simulink model "proyecto_4"  (R2021b)
settings: Solver=FixedStepDiscrete  StartTime=0.0  StopTime=Tsim  FixedStep=Tint  MaxStep=1e-6  RelTol=1e-6
InitFcn:
  | run init_fcn.m;
values from neighbouring files (symbols this model uses):
  C_init_v = 317    [init_fcn.m]
  C_load = 5e-2    (= 0.05)    [init_fcn.m]
  C_V = c_v * ro_air * volume_room    (= 220.63309632)    [init_fcn.m]
  Irr = 1000    [init_fcn.m]
  K_cond = Window_area * k_glass / esp    (= 158.4)    [init_fcn.m]
  L_s = 5e-3    (= 0.005)    [init_fcn.m]
  R_cuarto = 100    [init_fcn.m]
  shift = (180/3)/360 * Ts    (= 8.33333333333e-05)    [init_fcn.m]
  ss2 = c2d(ss2c, T_pred, 'tustin')    [init_fcn.m]
  T_ext = 15    [init_fcn.m]
  T_pred = Ts    (= 0.0005)    [init_fcn.m]
  Tint = 5e-5    (= 5e-05)    [init_fcn.m]
  Ts = 0.0005    [init_fcn.m]
  V_H4 = 300    [init_fcn.m]
  V_source = 230 * sqrt(2)    [init_fcn.m]
undefined symbols (not defined in the file or in its folder): DiscIntNeverNeededParam, F, K, Kobs, M, N, N2, Q, T_Enable, Temp_ref, Tsim, U0, X0
libraries: spsIGBTDiodeLib x17, spsVoltageMeasurementLib x11, simulink x8, spsCurrentMeasurementLib x8, slpidlib x6, spsSeriesRLCBranchLib x5, spsParallelRLCBranchLib x4, spsPVArrayLib x3, spsACVoltageSourceLib x1, spsDiodeLib x1, spspowerguiLib x1
(part 2 of 2)

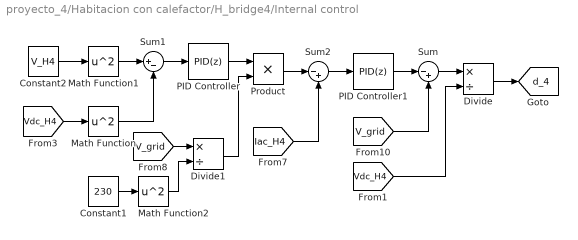
== system proyecto_4/Habitacion con calefactor/H_bridge4/Internal control ==
  Constant1 : Constant  Value=230
  Constant2 : Constant  Value=V_H4
  Divide : Product  Inputs=*/
  Divide1 : Product  Inputs=*/
  Math Function : Math  Operator=square  SaturateOnIntegerOverflow=on
  Math Function1 : Math  Operator=square  SaturateOnIntegerOverflow=on
  Math Function2 : Math  Operator=square  SaturateOnIntegerOverflow=on
  PID Controller : slpidlib/PID Controller  Controller=PID  Form=Parallel  TimeDomain=Discrete-time  UseExternalTs=off  SampleTime=Ts  IntegratorMethod=Forward Euler  FilterMethod=Forward Euler  ControllerParametersSource=internal  P=2  I=10  D=0  UseFilter=on  N=100  TunerSelectOption=Transfer Function Based (PID Tuner App)  InitialConditionSource=internal  InitialConditionForIntegrator=0  InitialConditionForFilter=0  DifferentiatorICPrevScaledInput=0  ExternalReset=none  TrackingMode=off  Kt=1  LimitOutput=off  SatLimitsSource=internal  UpperSaturationLimit=inf  LowerSaturationLimit=-inf  LinearizeAsGain=on  AntiWindupMode=none  Kb=1  POutMin=[]  POutMax=[]  IOutMin=[]  IOutMax=[]  DOutMin=[]  DOutMax=[]  NOutMin=[]  NOutMax=[]  SumOutMin=[]  SumOutMax=[]  SaturationOutMin=[]  SaturationOutMax=[]  PParamMin=[]  PParamMax=[]  IParamMin=[]  IParamMax=[]  DParamMin=[]  DParamMax=[]  NParamMin=[]  NParamMax=[]  KbParamMin=[]  KbParamMax=[]  KtParamMin=[]  KtParamMax=[]  KbOutMin=[]  KbOutMax=[]  KtOutMin=[]  KtOutMax=[]  IntegratorOutMin=[]  IntegratorOutMax=[]  FilterOutMin=[]  FilterOutMax=[]  SumI1OutMin=[]  SumI1OutMax=[]  SumI2OutMin=[]  SumI2OutMax=[]  SumI3OutMin=[]  SumI3OutMax=[]  SumI4OutMin=[]  SumI4OutMax=[]  SumDOutMin=[]  SumDOutMax=[]  DifferentiatorOutMin=[]  DifferentiatorOutMax=[]  FilterDiffOutCoefMin=[]  FilterDiffOutCoefMax=[]  ReciprocalOutMin=[]  ReciprocalOutMax=[]  SumDenOutMin=[]  SumDenOutMax=[]  SumNumOutMin=[]  SumNumOutMax=[]  DivideOutMin=[]  DivideOutMax=[]  UdiffTsProdOutMin=[]  UdiffTsProdOutMax=[]  NTsProdOutMin=[]  NTsProdOutMax=[]  UintegralTsProdOutMin=[]  UintegralTsProdOutMax=[]  UngainTsProdOutMin=[]  UngainTsProdOutMax=[]  IntegratorContinuousStateAttributes=''  IntegratorStateMustResolveToSignalObject=off  IntegratorRTWStateStorageClass=Auto  FilterContinuousStateAttributes=''  FilterStateMustResolveToSignalObject=off  FilterRTWStateStorageClass=Auto  ParallelPVariant=InternalParameters  IdealPVariant=Disabled  IVariant=InternalParameters  DVariant=InternalParameters  IntegratorVariant=Discrete  SatVariant=Disabled  AWVariant=Passthrough  PCopyVariant=Disabled  TRVariant=Disabled  FdbkBlocksVariant=Forward  IdealPFdbkVariant=Disabled  SatFdbkVariant=Disabled  DerivativeFilterVariant=ForwardEulerFilter  NVariant=InternalParameters  NCopyVariant=Disabled  FilterICVariant=InternalICsFilter  IntegratorICVariant=InternalICs  ExternalResetVariant=Disabled  TRSumVariant=Passthrough  SumFdbkVariant=Disabled  SumVariant=Sum_PID  TsampFilterVariant=InternalTs  TsampNgainVariant=Passthrough  TsampIntegralVariant=Passthrough  ExternalSaturationOutDataTypeStr=Inherit: Same as second input
  PID Controller1 : slpidlib/PID Controller  Controller=PID  Form=Parallel  TimeDomain=Discrete-time  UseExternalTs=off  SampleTime=Ts  IntegratorMethod=Forward Euler  FilterMethod=Forward Euler  ControllerParametersSource=internal  P=5  I=10  D=0  UseFilter=on  N=100  TunerSelectOption=Transfer Function Based (PID Tuner App)  InitialConditionSource=internal  InitialConditionForIntegrator=0  InitialConditionForFilter=0  DifferentiatorICPrevScaledInput=0  ExternalReset=none  TrackingMode=off  Kt=1  LimitOutput=off  SatLimitsSource=internal  UpperSaturationLimit=inf  LowerSaturationLimit=-inf  LinearizeAsGain=on  AntiWindupMode=none  Kb=1  POutMin=[]  POutMax=[]  IOutMin=[]  IOutMax=[]  DOutMin=[]  DOutMax=[]  NOutMin=[]  NOutMax=[]  SumOutMin=[]  SumOutMax=[]  SaturationOutMin=[]  SaturationOutMax=[]  PParamMin=[]  PParamMax=[]  IParamMin=[]  IParamMax=[]  DParamMin=[]  DParamMax=[]  NParamMin=[]  NParamMax=[]  KbParamMin=[]  KbParamMax=[]  KtParamMin=[]  KtParamMax=[]  KbOutMin=[]  KbOutMax=[]  KtOutMin=[]  KtOutMax=[]  IntegratorOutMin=[]  IntegratorOutMax=[]  FilterOutMin=[]  FilterOutMax=[]  SumI1OutMin=[]  SumI1OutMax=[]  SumI2OutMin=[]  SumI2OutMax=[]  SumI3OutMin=[]  SumI3OutMax=[]  SumI4OutMin=[]  SumI4OutMax=[]  SumDOutMin=[]  SumDOutMax=[]  DifferentiatorOutMin=[]  DifferentiatorOutMax=[]  FilterDiffOutCoefMin=[]  FilterDiffOutCoefMax=[]  ReciprocalOutMin=[]  ReciprocalOutMax=[]  SumDenOutMin=[]  SumDenOutMax=[]  SumNumOutMin=[]  SumNumOutMax=[]  DivideOutMin=[]  DivideOutMax=[]  UdiffTsProdOutMin=[]  UdiffTsProdOutMax=[]  NTsProdOutMin=[]  NTsProdOutMax=[]  UintegralTsProdOutMin=[]  UintegralTsProdOutMax=[]  UngainTsProdOutMin=[]  UngainTsProdOutMax=[]  IntegratorContinuousStateAttributes=''  IntegratorStateMustResolveToSignalObject=off  IntegratorRTWStateStorageClass=Auto  FilterContinuousStateAttributes=''  FilterStateMustResolveToSignalObject=off  FilterRTWStateStorageClass=Auto  ParallelPVariant=InternalParameters  IdealPVariant=Disabled  IVariant=InternalParameters  DVariant=InternalParameters  IntegratorVariant=Discrete  SatVariant=Disabled  AWVariant=Passthrough  PCopyVariant=Disabled  TRVariant=Disabled  FdbkBlocksVariant=Forward  IdealPFdbkVariant=Disabled  SatFdbkVariant=Disabled  DerivativeFilterVariant=ForwardEulerFilter  NVariant=InternalParameters  NCopyVariant=Disabled  FilterICVariant=InternalICsFilter  IntegratorICVariant=InternalICs  ExternalResetVariant=Disabled  TRSumVariant=Passthrough  SumFdbkVariant=Disabled  SumVariant=Sum_PID  TsampFilterVariant=InternalTs  TsampNgainVariant=Passthrough  TsampIntegralVariant=Passthrough  ExternalSaturationOutDataTypeStr=Inherit: Same as second input
  Product : Product
  Sum : Sum  Inputs=|-+
  Sum1 : Sum  Inputs=|+-
  Sum2 : Sum  Inputs=|-+
  tag scope: d_4=global
  wires:
  Divide/1 -> [d_4]
  Math Function1/1 -> Sum1/1
  [Iac_H4] -> Sum2/2
  Sum1/1 -> PID Controller/1
  Math Function/1 -> Sum1/2
  PID Controller1/1 -> Sum/1
  [Vdc_H4] -> Math Function/1
  PID Controller/1 -> Product/1
  Divide1/1 -> Product/2
  [V_grid] -> Sum/2
  Sum2/1 -> PID Controller1/1
  Sum/1 -> Divide/1
  [Vdc_H4] -> Divide/2
  Constant1/1 -> Math Function2/1
  [V_grid] -> Divide1/1
  Math Function2/1 -> Divide1/2
  Product/1 -> Sum2/1
  Constant2/1 -> Math Function1/1

== system proyecto_4/Habitacion con calefactor/H_bridge4/Measurements ==
  Current Measurement : spsCurrentMeasurementLib/Current Measurement  PhasorSimulation=off  OutputType=Complex  PSBequivalent=0
  V : spsVoltageMeasurementLib/Voltage Measurement  PhasorSimulation=off  OutputType=Complex  PSBequivalent=0
  in + : PMIOPort  Side=Left
  - : PMIOPort  Port=2  Side=Left
  out + : PMIOPort  Port=3  Side=Right
  -- : PMIOPort  Port=4  Side=Right
  tag scope: Iac_H4=global, Vac_H4=global
  wires:
  V/1 -> [Vac_H4]
  Current Measurement/1 -> [Iac_H4]
  connections:
  V/LConn2 -- --/RConn1 -- -/RConn1
  V/LConn1 -- Current Measurement/RConn1 -- out +/RConn1
  Current Measurement/LConn1 -- in +/RConn1

== system proyecto_4/Habitacion con calefactor/H_bridge4/Measurements1 ==
  Current Measurement : spsCurrentMeasurementLib/Current Measurement  PhasorSimulation=off  OutputType=Complex  PSBequivalent=0
  V : spsVoltageMeasurementLib/Voltage Measurement  PhasorSimulation=off  OutputType=Complex  PSBequivalent=0
  i + : PMIOPort  Side=Left
  i - : PMIOPort  Port=2  Side=Left
  o + : PMIOPort  Port=3  Side=Right
  o- : PMIOPort  Port=4  Side=Right
  tag scope: Idc_H4=global, Vdc_H4=global
  wires:
  V/1 -> [Vdc_H4]
  Current Measurement/1 -> [Idc_H4]
  connections:
  o-/RConn1 -- i -/RConn1 -- V/LConn2
  V/LConn1 -- o +/RConn1 -- Current Measurement/LConn1
  Current Measurement/RConn1 -- i +/RConn1

== system proyecto_4/H_bridge1/H_basic/Modulator2/Restriccion ==
  In1 : Inport
  In2 : Inport  Port=2
  Logical Operator1 : Logic  Operator=NOT  AllPortsSameDT=off  OutDataTypeStr=boolean
  Logical Operator2 : Logic  Operator=NOT  AllPortsSameDT=off  OutDataTypeStr=boolean
  Out1 : Outport
  Out2 : Outport  Port=2
  Out3 : Outport  Port=3
  Out4 : Outport  Port=4
  wires:
  In1/1 -> Out1/1, Logical Operator1/1
  In2/1 -> Out3/1, Logical Operator2/1
  Logical Operator2/1 -> Out4/1
  Logical Operator1/1 -> Out2/1

== system proyecto_4/H_bridge1/H_basic/Modulator2/Unipolar ==
  Duty : Inport
  Triag : Inport  Port=2
  Gain : Gain  Gain=-1
  Relational Operator : RelationalOperator  OutDataTypeStr=boolean  RndMeth=Simplest
  Relational Operator1 : RelationalOperator  OutDataTypeStr=boolean  RndMeth=Simplest
  Out1 : Outport
  Out2 : Outport  Port=2
  wires:
  Relational Operator/1 -> Out1/1
  Triag/1 -> Relational Operator/2, Gain/1
  Duty/1 -> Relational Operator1/2, Relational Operator/1
  Relational Operator1/1 -> Out2/1
  Gain/1 -> Relational Operator1/1

== system proyecto_4/H_bridge2/H_basic/Modulator2/Restriccion ==
  In1 : Inport
  In2 : Inport  Port=2
  Logical Operator1 : Logic  Operator=NOT  AllPortsSameDT=off  OutDataTypeStr=boolean
  Logical Operator2 : Logic  Operator=NOT  AllPortsSameDT=off  OutDataTypeStr=boolean
  Out1 : Outport
  Out2 : Outport  Port=2
  Out3 : Outport  Port=3
  Out4 : Outport  Port=4
  wires:
  In1/1 -> Out1/1, Logical Operator1/1
  In2/1 -> Out3/1, Logical Operator2/1
  Logical Operator2/1 -> Out4/1
  Logical Operator1/1 -> Out2/1

== system proyecto_4/H_bridge2/H_basic/Modulator2/Unipolar ==
  Duty : Inport
  Triag : Inport  Port=2
  Gain : Gain  Gain=-1
  Relational Operator : RelationalOperator  OutDataTypeStr=boolean  RndMeth=Simplest
  Relational Operator1 : RelationalOperator  OutDataTypeStr=boolean  RndMeth=Simplest
  Out1 : Outport
  Out2 : Outport  Port=2
  wires:
  Relational Operator/1 -> Out1/1
  Triag/1 -> Relational Operator/2, Gain/1
  Duty/1 -> Relational Operator1/2, Relational Operator/1
  Relational Operator1/1 -> Out2/1
  Gain/1 -> Relational Operator1/1

== system proyecto_4/H_bridge3/H_basic/Modulator2/Restriccion ==
  In1 : Inport
  In2 : Inport  Port=2
  Logical Operator1 : Logic  Operator=NOT  AllPortsSameDT=off  OutDataTypeStr=boolean
  Logical Operator2 : Logic  Operator=NOT  AllPortsSameDT=off  OutDataTypeStr=boolean
  Out1 : Outport
  Out2 : Outport  Port=2
  Out3 : Outport  Port=3
  Out4 : Outport  Port=4
  wires:
  In1/1 -> Out1/1, Logical Operator1/1
  In2/1 -> Out3/1, Logical Operator2/1
  Logical Operator2/1 -> Out4/1
  Logical Operator1/1 -> Out2/1

== system proyecto_4/H_bridge3/H_basic/Modulator2/Unipolar ==
  Duty : Inport
  Triag : Inport  Port=2
  Gain : Gain  Gain=-1
  Relational Operator : RelationalOperator  OutDataTypeStr=boolean  RndMeth=Simplest
  Relational Operator1 : RelationalOperator  OutDataTypeStr=boolean  RndMeth=Simplest
  Out1 : Outport
  Out2 : Outport  Port=2
  wires:
  Relational Operator/1 -> Out1/1
  Triag/1 -> Relational Operator/2, Gain/1
  Duty/1 -> Relational Operator1/2, Relational Operator/1
  Relational Operator1/1 -> Out2/1
  Gain/1 -> Relational Operator1/1

== system proyecto_4/Habitacion con calefactor/H_bridge4/H_basic/Modulator2 ==
  Mux : Mux
  Restriccion : Subsystem
  Transport Delay : TransportDelay  DelayTime=shift
  Unipolar : Subsystem
  Out1 : Outport
  wires:
  Restriccion/1(Out1) -> Mux/1
  [d_4] -> Unipolar/1(Duty)
  Mux/1 -> Out1/1
  Restriccion/4(Out4) -> Mux/4
  Unipolar/1(Out1) -> Restriccion/1(In1)
  Restriccion/3(Out3) -> Mux/3
  Unipolar/2(Out2) -> Restriccion/2(In2)
  Restriccion/2(Out2) -> Mux/2
  [Triag] -> Transport Delay/1
  Transport Delay/1 -> Unipolar/2(Triag)

== system proyecto_4/Habitacion con calefactor/H_bridge4/H_basic/Modulator2/Restriccion ==
  In1 : Inport
  In2 : Inport  Port=2
  Logical Operator1 : Logic  Operator=NOT  AllPortsSameDT=off  OutDataTypeStr=boolean
  Logical Operator2 : Logic  Operator=NOT  AllPortsSameDT=off  OutDataTypeStr=boolean
  Out1 : Outport
  Out2 : Outport  Port=2
  Out3 : Outport  Port=3
  Out4 : Outport  Port=4
  wires:
  In1/1 -> Out1/1, Logical Operator1/1
  In2/1 -> Out3/1, Logical Operator2/1
  Logical Operator2/1 -> Out4/1
  Logical Operator1/1 -> Out2/1

== system proyecto_4/Habitacion con calefactor/H_bridge4/H_basic/Modulator2/Unipolar ==
  Duty : Inport
  Triag : Inport  Port=2
  Gain : Gain  Gain=-1
  Relational Operator : RelationalOperator  OutDataTypeStr=boolean  RndMeth=Simplest
  Relational Operator1 : RelationalOperator  OutDataTypeStr=boolean  RndMeth=Simplest
  Out1 : Outport
  Out2 : Outport  Port=2
  wires:
  Relational Operator/1 -> Out1/1
  Triag/1 -> Relational Operator/2, Gain/1
  Duty/1 -> Relational Operator1/2, Relational Operator/1
  Relational Operator1/1 -> Out2/1
  Gain/1 -> Relational Operator1/1
